simulink model "Six_DoF_Plot_Test"  (R2020a)
settings: Solver=VariableStepAuto  StartTime=0.0  StopTime=40  RelTol=1e-3
InitFcn:
  | drone_param
StartFcn:
  | drone_param
undefined symbols (not defined in the file or in its folder): drawDrone, P
libraries: simulink x6
ContinueFcn:
  | FT2frfl
settings Model: Creator=sadam  LastModifiedBy=Adam
settings DataIOCC: ReturnWorkspaceOutputs=off
settings DebuggingCC: ArithmeticOperatorsInVariantConditions=warning
settings SFSimCC: SimUseLocalCustomCode=off  CustomCodeUndefinedFunction=UseInterfaceOnly
settings RTWCC: RTWUseLocalCustomCode=off

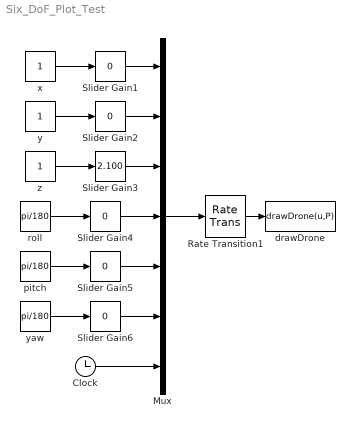
== system Six_DoF_Plot_Test ==
  Clock : Clock
  Mux : Mux  Inputs=7
  Rate Transition1 : RateTransition  OutPortSampleTime=P.t_plot
  Slider Gain{1..2,4..6} (5 alike) : simulink/Math Operations/Slider Gain  gain=0  low=-5  high=5
  Slider Gain3 : simulink/Math Operations/Slider Gain  gain=2.100  low=-5  high=5
  drawDrone : MATLABFcn  MATLABFcn=drawDrone(u,P)  OutputDimensions=0
  pitch : Constant  Value=pi/180
  roll : Constant  Value=pi/180
  x : Constant
  y : Constant
  yaw : Constant  Value=pi/180
  z : Constant
  wires:
  Mux/1 -> Rate Transition1/1
  Rate Transition1/1 -> drawDrone/1
  x/1 -> Slider Gain1/1
  y/1 -> Slider Gain2/1
  z/1 -> Slider Gain3/1
  Slider Gain1/1 -> Mux/1
  Slider Gain2/1 -> Mux/2
  Slider Gain3/1 -> Mux/3
  yaw/1 -> Slider Gain6/1
  roll/1 -> Slider Gain4/1
  pitch/1 -> Slider Gain5/1
  Slider Gain4/1 -> Mux/4
  Slider Gain5/1 -> Mux/5
  Slider Gain6/1 -> Mux/6
  Clock/1 -> Mux/7
